simulink model "closedloop"  (R2023a)
settings: Solver=VariableStepAuto  StartTime=0.0  StopTime=21  RelTol=1e-3
values from neighbouring files (symbols this model uses):
  sampling_time = 1 / 50    (= 0.02)    [controller_design.m]    (also in dtime_data.m = 1 / sampling_frequencies(i); nlinear_data.m)
  time_delay = mean(diffs)    [vision_delay.m]
undefined symbols (not defined in the file or in its folder): c_a, c_b, c_disc_a, c_disc_b, DiscIntNeverNeededParam, gyro_sigma_drift, init, sys_a, sys_b, theta_l_init, V_bar, vision_fps, wave_amplitude, wave_offset, wave_period, x2_bar
settings Model: Creator=yunzh  LastModifiedBy=yunzh

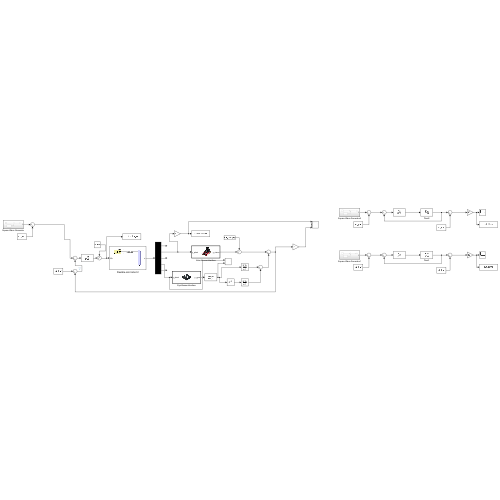
[thumbnail: Simulink's stored preview of the top-level diagram]
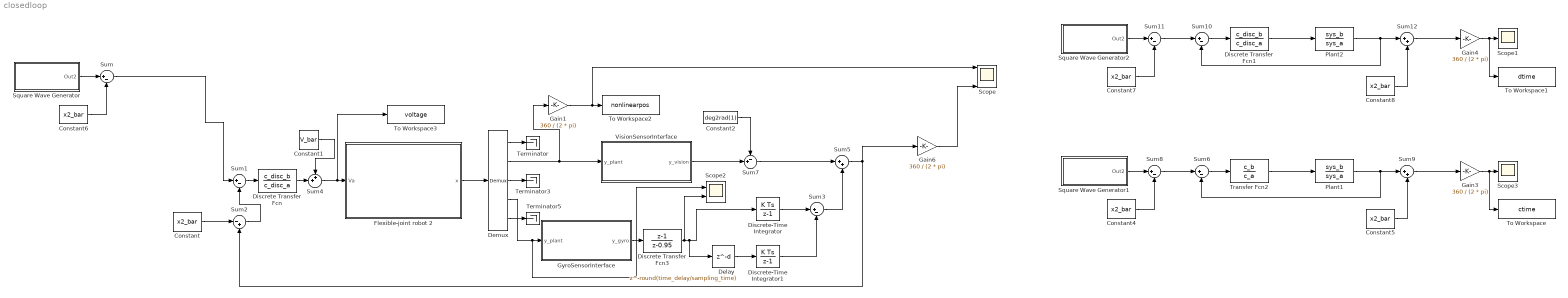
== system closedloop ==
  Constant{,4..8} (6 alike) : Constant  Value=x2_bar
  Constant1 : Constant  Value=V_bar
  Constant2 : Constant  Value=deg2rad(1)
  Delay : Delay  DelayLength=round(time_delay/sampling_time)  InitialCondition=0
  Demux : Demux  Outputs=5
  Discrete Transfer Fcn : DiscreteTransferFcn  Numerator=c_disc_b  Denominator=c_disc_a  SampleTime=sampling_time
  Discrete Transfer Fcn1 : DiscreteTransferFcn  Numerator=c_disc_b  Denominator=c_disc_a  SampleTime=sampling_time
  Discrete Transfer Fcn3 : DiscreteTransferFcn  Numerator=[1 -1]  Denominator=[1 -0.95]  SampleTime=sampling_time
  Discrete-Time Integrator : DiscreteIntegrator  InitialCondition=theta_l_init  SampleTime=-1  ICPrevOutput=DiscIntNeverNeededParam  ICPrevScaledInput=DiscIntNeverNeededParam
  Discrete-Time Integrator1 : DiscreteIntegrator  InitialCondition=theta_l_init  SampleTime=-1  ICPrevOutput=DiscIntNeverNeededParam  ICPrevScaledInput=DiscIntNeverNeededParam
  Flexible-joint robot 2 : Subsystem
      mask Display: image('$imagefile'); % Use "Edit Image" on toolstrip to change.
  Gain{1,3..4,6} (4 alike) : Gain  Gain=360 / (2 * pi)
  GyroSensorInterface : Subsystem  TreatAsAtomicUnit=on
      mask Display: image('$imagefile'); % Use "Edit Image" on toolstrip to change.
  Plant1 : TransferFcn  Numerator=sys_b  Denominator=sys_a
  Plant2 : TransferFcn  Numerator=sys_b  Denominator=sys_a
  Scope : Scope  NumInputPorts=4
  Scope1 : Scope
  Scope2 : Scope  NumInputPorts=2
  Scope3 : Scope
  Square Wave Generator : Subsystem
  Square Wave Generator1 : Subsystem
  Square Wave Generator2 : Subsystem
  Sum{,1,3,6,8,10..11} (7 alike) : Sum  Inputs=|+-
  Sum12 : Sum  Inputs=|++
  Sum2 : Sum  Inputs=|-+
  Sum4 : Sum  Inputs=++|
  Sum5 : Sum  Inputs=|++
  Sum7 : Sum  Inputs=-+|
  Sum9 : Sum  Inputs=|++
  Terminator : Terminator
  Terminator3 : Terminator
  Terminator5 : Terminator
  To Workspace : ToWorkspace  VariableName=ctime  SaveFormat=Timeseries  SampleTime=-1
  To Workspace1 : ToWorkspace  VariableName=dtime  SaveFormat=Timeseries  SampleTime=-1
  To Workspace2 : ToWorkspace  VariableName=nonlinearpos  SaveFormat=Timeseries  SampleTime=-1
  To Workspace3 : ToWorkspace  VariableName=voltage  SaveFormat=Timeseries  SampleTime=-1
  Transfer Fcn2 : TransferFcn  Numerator=c_b  Denominator=c_a
  VisionSensorInterface : Subsystem  TreatAsAtomicUnit=on
      mask Display: image('$imagefile'); % Use "Edit Image" on toolstrip to change.
  wires:
  Flexible-joint robot 2/1(x) -> Demux/1
  Demux/5 -> Terminator5/1
  Demux/3 -> Terminator3/1
  Demux/1 -> Terminator/1
  Gain1/1 -> Scope/1, To Workspace2/1
  Constant/1 -> Sum2/1
  Sum2/1 -> Sum1/2
  Discrete Transfer Fcn/1 -> Sum4/2
  Sum4/1 -> To Workspace3/1, Flexible-joint robot 2/1(Va)
  Constant1/1 -> Sum4/1
  Square Wave Generator/1(Out2) -> Sum/1
  Sum/1 -> Sum1/1
  Constant6/1 -> Sum/2
  Demux/2 -> VisionSensorInterface/1(y_plant), Gain1/1
  Plant1/1 -> Sum9/1, Sum6/2
  Sum6/1 -> Transfer Fcn2/1
  Transfer Fcn2/1 -> Plant1/1
  Sum1/1 -> Discrete Transfer Fcn/1
  Square Wave Generator1/1(Out2) -> Sum8/1
  Constant4/1 -> Sum8/2
  Sum8/1 -> Sum6/1
  Gain3/1 -> To Workspace/1, Scope3/1
  Sum9/1 -> Gain3/1
  Constant5/1 -> Sum9/2
  Gain4/1 -> To Workspace1/1, Scope1/1
  Square Wave Generator2/1(Out2) -> Sum11/1
  Discrete Transfer Fcn1/1 -> Plant2/1
  Plant2/1 -> Sum12/1, Sum10/2
  Sum10/1 -> Discrete Transfer Fcn1/1
  Constant8/1 -> Sum12/2
  Sum11/1 -> Sum10/1
  Sum12/1 -> Gain4/1
  Constant7/1 -> Sum11/2
  GyroSensorInterface/1(y_gyro) -> Discrete Transfer Fcn3/1
  Delay/1 -> Discrete-Time Integrator1/1
  Discrete-Time Integrator1/1 -> Sum3/2
  Discrete-Time Integrator/1 -> Sum3/1
  Sum5/1 -> Gain6/1, Sum2/2
  VisionSensorInterface/1(y_vision) -> Sum7/2
  Sum7/1 -> Sum5/1
  Constant2/1 -> Sum7/1
  Demux/4 -> Scope2/1, GyroSensorInterface/1(y_plant)
  Gain6/1 -> Scope/4
  Discrete Transfer Fcn3/1 -> Scope2/2, Delay/1, Discrete-Time Integrator/1
  Sum3/1 -> Sum5/2

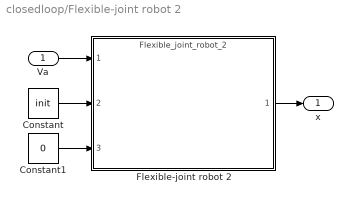
== system closedloop/Flexible-joint robot 2 ==
  Va : Inport
  Constant : Constant  Value=init
  Constant1 : Constant  Value=0
  Flexible-joint robot 2 : ModelReference  ModelNameDialog=Flexible_joint_robot_2  ModelReferenceVersion=1.65  CopyOfModelProtected=on
  x : Outport
  wires:
  Va/1 -> Flexible-joint robot 2/1
  Constant1/1 -> Flexible-joint robot 2/3
  Constant/1 -> Flexible-joint robot 2/2
  Flexible-joint robot 2/1 -> x/1

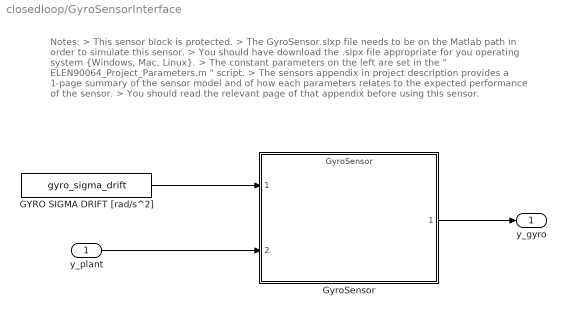
== system closedloop/GyroSensorInterface ==
  note: Notes:
      | > This sensor block is protected.
      | > The GyroSensor.slxp file needs to be on the Matlab path in order to simulate this sensor.
      | > You should have download the .slpx file appropriate for you operating system {Windows, Mac, Linux}.
      | > The constant parameters on the left are set in the " ELEN90064_Project_Parameters.m " script.
      | > The sensors appendix in project description provides a 1-page summary of the sensor model and of how each parameters relates to the expected performance of the sensor.
      | > You should read the relevant page of that appendix before using this sensor.
  y_plant : Inport
  GYRO SIGMA DRIFT [rad/s^2] : Constant  Value=gyro_sigma_drift
  GyroSensor : ModelReference  ModelNameDialog=GyroSensor.slxp  ModelReferenceVersion=1.18  CopyOfModelProtected=on
  y_gyro : Outport
  wires:
  GYRO SIGMA DRIFT [rad/s^2]/1 -> GyroSensor/1
  y_plant/1 -> GyroSensor/2
  GyroSensor/1 -> y_gyro/1

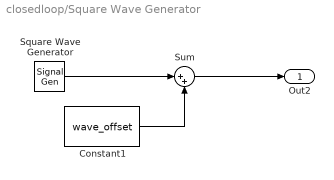
== system closedloop/Square Wave Generator ==
  Constant1 : Constant  Value=wave_offset
  Square Wave Generator : SignalGenerator  WaveForm=square  Amplitude=wave_amplitude  Frequency=1 / wave_period
  Sum : Sum  Inputs=|++
  Out2 : Outport
  wires:
  Square Wave Generator/1 -> Sum/1
  Constant1/1 -> Sum/2
  Sum/1 -> Out2/1

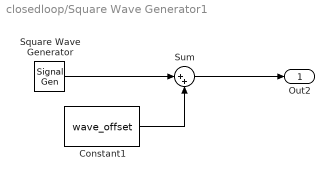
== system closedloop/Square Wave Generator1 ==
  Constant1 : Constant  Value=wave_offset
  Square Wave Generator : SignalGenerator  WaveForm=square  Amplitude=wave_amplitude  Frequency=1 / wave_period
  Sum : Sum  Inputs=|++
  Out2 : Outport
  wires:
  Square Wave Generator/1 -> Sum/1
  Constant1/1 -> Sum/2
  Sum/1 -> Out2/1

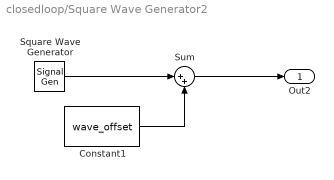
== system closedloop/Square Wave Generator2 ==
  Constant1 : Constant  Value=wave_offset
  Square Wave Generator : SignalGenerator  WaveForm=square  Amplitude=wave_amplitude  Frequency=1 / wave_period
  Sum : Sum  Inputs=|++
  Out2 : Outport
  wires:
  Square Wave Generator/1 -> Sum/1
  Constant1/1 -> Sum/2
  Sum/1 -> Out2/1

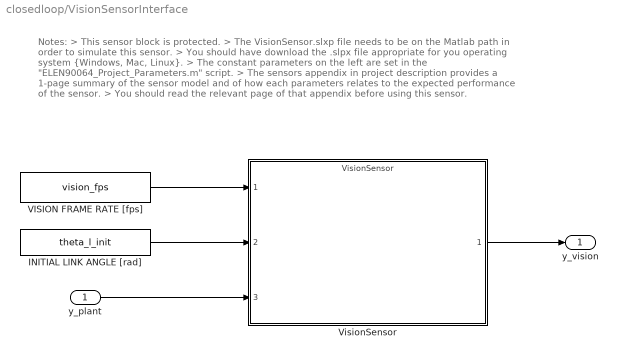
== system closedloop/VisionSensorInterface ==
  note: Notes:
      | > This sensor block is protected.
      | > The VisionSensor.slxp file needs to be on the Matlab path in order to simulate this sensor.
      | > You should have download the .slpx file appropriate for you operating system {Windows, Mac, Linux}.
      | > The constant parameters on the left are set in the "ELEN90064_Project_Parameters.m" script.
      | > The sensors appendix in project description provides a 1-page summary of the sensor model and of how each parameters relates to the expected performance of the sensor.
      | > You should read the relevant page of that appendix before using this sensor.
  y_plant : Inport
  INITIAL LINK ANGLE [rad] : Constant  Value=theta_l_init
  VISION FRAME RATE [fps] : Constant  Value=vision_fps
  VisionSensor : ModelReference  ModelNameDialog=VisionSensor.slxp  ModelReferenceVersion=1.19  CopyOfModelProtected=on
  y_vision : Outport
  wires:
  VISION FRAME RATE [fps]/1 -> VisionSensor/1
  INITIAL LINK ANGLE [rad]/1 -> VisionSensor/2
  y_plant/1 -> VisionSensor/3
  VisionSensor/1 -> y_vision/1
